simulink model "stateflow_on_arduino"  (R2020b)
settings: Solver=FixedStepAuto  StartTime=0.0  StopTime=inf  FixedStep=h  RelTol=1e-3
undefined symbols (not defined in the file): h
libraries: arduinolib x5
settings Model: SILPILModeSetting=veronly  ExtModeTrigDuration=2  Creator=natha  LastModifiedBy=natha
settings OptimizationCC: EnhancedBackFolding=on  PassReuseOutputArgsAs=Individual arguments  ZeroExternalMemoryAtStartup=off  ZeroInternalMemoryAtStartup=off  MaxStackSize=64  OptimizeBlockOrder=speed  DifferentSizesBufferReuse=on  OptimizationCustomize=off  EfficientTunableParamExpr=on
settings DebuggingCC: ParameterTunabilityLossMsg=error
settings HardwareCC: ProdBitPerInt=16  ProdBitPerPointer=16  ProdBitPerSizeT=16  ProdBitPerPtrDiffT=16  ProdLargestAtomicFloat=None  ProdWordSize=8  ProdHWDeviceType=Atmel->AVR  UseEmbeddedCoderFeatures=off  UseSimulinkCoderFeatures=off
settings SFSimCC: MATLABDynamicMemAlloc=off
settings RTWCC: Description=Embedded Coder  SystemTargetFile=ert.tlc  HardwareBoard=Arduino Mega 2560  TemplateMakefile=ert_default_tmf  Toolchain=Arduino AVR
settings CodeAppCC: ForceParamTrailComments=on  IgnoreCustomStorageClasses=off  OperatorAnnotations=on  SimulinkDataObjDesc=on  SFDataObjDesc=on  MangleLength=10  InsertBlockDesc=on
settings ERTTargetCC: SupportContinuousTime=on  SupportNonInlinedSFcns=on  SupportVariableSizeSignals=on  ExtModeStaticAllocSize=2048

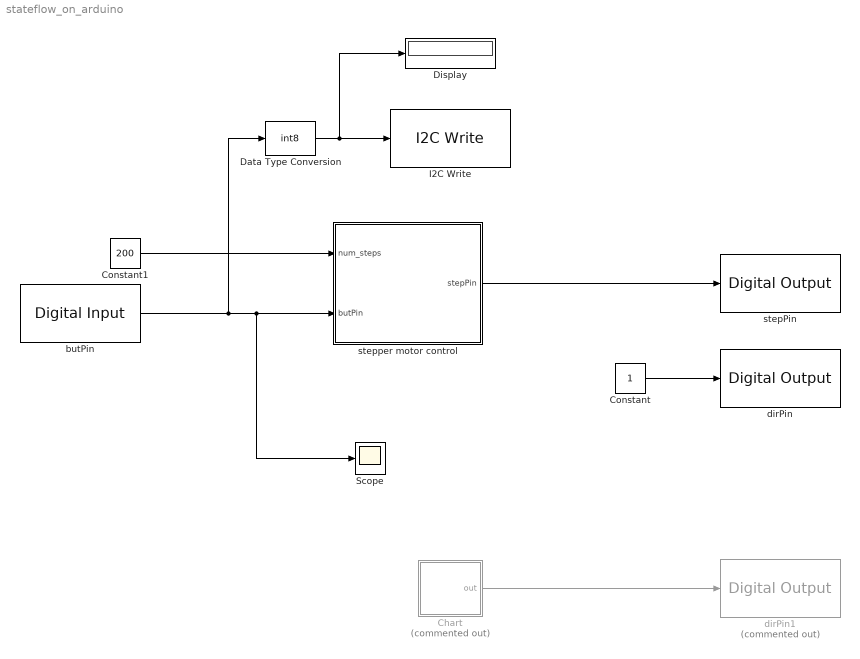
== system stateflow_on_arduino ==
  Chart : Stateflow chart  Commented=on  TreatAsAtomicUnit=on
  Constant : Constant
  Constant1 : Constant  Value=200
  Data Type Conversion : DataTypeConversion  OutDataTypeStr=int8
  Display : Display
  I2C Write : arduinolib/I2C Write  I2CModule=0  Mode=Master  SlaveAddress=1  SlaveByteOrder=BigEndian  Direction=Transmitter  RegisterAddressMode=off  RegisterAddress=0  SlaveDataType=uint8  DataLength=1  NoAck=off  RepeatedStart=off  OutputStatus=off  blockPlatform=ARDUINO
      settings: SourceProductBaseCode=ARDUINO
  Scope : Scope
  butPin : arduinolib/Digital Input  pinNumber=8  mode=Default  Direction=input  SampleTime=h  blockPlatform=arduino
  dirPin : arduinolib/Digital Output  pinNumber=4  Direction=output  blockPlatform=arduino
  dirPin1 : arduinolib/Digital Output  Commented=on  pinNumber=10  Direction=output  blockPlatform=arduino
  stepPin : arduinolib/Digital Output  pinNumber=3  Direction=output  blockPlatform=arduino
  stepper motor control : Stateflow chart  TreatAsAtomicUnit=on
  wires:
  Constant/1 -> dirPin/1
  butPin/1 -> Data Type Conversion/1, Scope/1, stepper motor control/2(butPin)
  stepper motor control/1(stepPin) -> stepPin/1
  Constant1/1 -> stepper motor control/1(num_steps)
  Chart/1(out) -> dirPin1/1
  Data Type Conversion/1 -> Display/1, I2C Write/1

== stateflow chart stateflow_on_arduino/Chart ==
  state on
    entry: out=1;
  state off
    entry: out=0;
  (default) -> on
  off -> on : after(1,sec)
  on -> off : after(1,sec)
  data: out output

== stateflow chart stateflow_on_arduino/stepper motor control ==
  state stepper_motor_inactive
  state stepper_motor_on
    state low
      entry: stepPin=0;
    state high
      entry: stepPin=1;
    high -> low : after(3,msec)
    low -> high [order 2] : after(3,msec){i=i+1;}
  (default) -> stepper_motor_inactive
  low -> stepper_motor_inactive [order 1] : [i==num_steps]
  stepper_motor_inactive -> high [order 2] : after(5,sec){i=1;}
  stepper_motor_inactive -> high [order 1] : [butPin==1]{i=1;}
  data: num_steps input; i local; stepPin output; butPin input size=[1 1]
